simulink model "SimscapeCrane_ClosedLoop"  (R2017a)
settings: Solver=ode15s  StartTime=0.0  StopTime=20  RelTol=1e-3  EnableMultiTasking=on
model workspace: external: MAT-File workspace.mat (data not in the file)
values from neighbouring files (symbols this model uses):
  m = 0.47    [workspace.mat]
  MR = 1.71    [workspace.mat]
  N = 30    [FunctionTemplate.m]    (also in mySetup.m; testMyDesign_Linear.m = ceil(T/Ts))
  Ts = 1/20    (= 0.05)    [FunctionTemplate.m]    (also in mySetup.m; testMyDesign.m; testMyDesign_Linear.m; workspace.mat)
  TxBreak = 0    [workspace.mat]
  TxCoulomb = 3.7489    [workspace.mat]
  TxTrans = 0.02    [workspace.mat]
  TxVisc = 58.085    [workspace.mat]
  TyBreak = 0    [workspace.mat]
  TyCoulomb = 2.674    [workspace.mat]
  TyTrans = 0.02    [workspace.mat]
  TzBreak = 0    [workspace.mat]
  TzCoulomb = 6.1    [workspace.mat]
  TzTrans = 0.2    [workspace.mat]
  xRange = [0 0.52]    [workspace.mat]
  xZero = testShape.start(1,1)    [testMyDesign.m]    (also in testMyDesign_Linear.m; workspace.mat = 0.0353553390593)
  yRange = [0 0.62]    [workspace.mat]
  yZero = testShape.start(1,2)    [testMyDesign.m]    (also in testMyDesign_Linear.m; workspace.mat = 0.0707106781187)
  zRange = [0.17 0.8]    [workspace.mat]
  zZero = 0.47    [workspace.mat]
undefined symbols (not defined in the file or in its folder): X, Y, Z
undefined symbols (not defined in the file): M, param, TorqueMultX, TorqueMultY, TorqueMultZ, TyVisc, TzVisc
libraries: sm_lib x146, fl_lib x62, nesl_utility x24, elec_lib x9, simulink x6, sm_double_wishbone_suspension_lib x4, sharedtransform x1
(part 1 of 14)
settings Model: Creator=jsustare  LastModifiedBy=ferra
settings SolverCC: MaxConsecutiveMinStep=10
settings DataIOCC: SaveFormat=StructureWithTime
settings OptimizationCC: LifeSpan=inf
settings DebuggingCC: AllowSymbolicDim=off  SFUnexpectedBacktrackingDiag=warning  SFNoUnconditionalDefaultTransitionDiag=warning  SFExecutionAtInitializationDiag=none
settings ModelReferenceCC: PropagateSignalLabelsOutOfModel=off
settings GRTTargetCC: TargetLangStandard=C89/C90 (ANSI)
settings ConfigComp: CovMetricSettings=dw  CovHtmlReporting=on  CovSaveCumulativeToWorkspaceVar=on  CovSaveSingleToWorkspaceVar=on  CovExternalEMLEnable=off
settings ConfigurationSet: Description=SimMechanics 2G

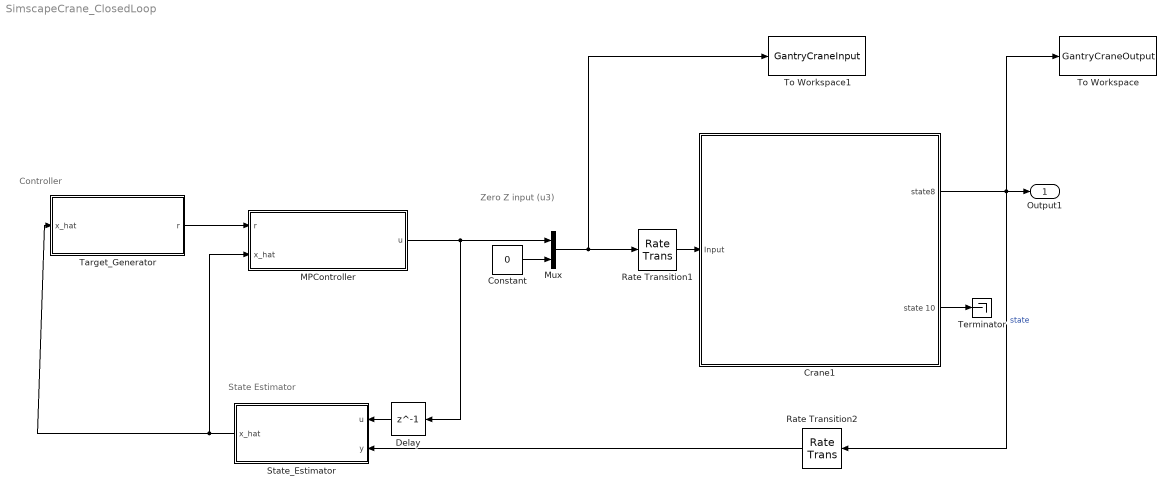
== system SimscapeCrane_ClosedLoop ==
  note: Controller
  note: Zero Z input (u3)
  note: State Estimator
  Constant : Constant  Value=0
  Crane1 : Subsystem  mask{penduMass=m, cartMass=M, MR=MR, xRange=xRange, yRange=yRange, zRange=zRange, xZero=xZero, yZero=yZero, zZero=zZero, TxBreak=TxBreak, TxCoulomb=TxCoulomb, TxVisc=TxVisc, TxTrans=TxTrans, TyBreak=TyBreak, TyCoulomb=TyCoulomb, TyVisc=TyVisc, TyTrans=TyTrans, TzBreak=TzBreak, TzCoulomb=TzCoulomb, TzVisc=TzVisc, TzTrans=TzTrans, Ux=TorqueMultX, Uy=TorqueMultY, Uz=TorqueMultZ}
      mask prompts: penduMass "Pendulum Mass (Kg)"; cartMass "Mass of the cart (Kg)"; MR "Mass of the rail (Kg)"; TxBreak "BreakAwayFriction"; TxCoulomb "Coulomb Friction"; TxVisc "Viscous friction"; TxTrans "Transition coeff"; TyBreak "BreakAwayFriction"; TyCoulomb "Coulomb Friction"; TyVisc "Viscous friction"; TyTrans "Transition coeff"; TzBreak "BreakAwayFriction"; TzCoulomb "Coulomb Friction"; TzVisc "Viscous friction"; TzTrans "Transition coeff"; Ux "Rail motor multiplier (X)"; Uy "Cart motor multiplier (Y)"; Uz "String motor multiplier (Z)"
      mask init:
      | %mass lowSat
      | penduMass=max(penduMass,1e-3);
      | cartMass=max(cartMass,1e-3);
      | MR=max(MR,1e-3);
      | 
      | %zeros saturated
      | xZero=max(xZero,xRange(1));
      | xZero=min(xZero,xRange(2));
      | 
      | yZero=max(yZero,yRange(1));
      | yZero=min(yZero,yRange(2));
      | 
      | zZero=max(zZero,zRange(1));
      | zZero=min(zZero,zRange(2));
      mask DialogControl DescGroupVar Prompt: 3D Crane Simscape model
      mask Display:
